simulink model "Angle_from_mpu6050_example"  (R2020b)
settings: Solver=FixedStepAuto  StartTime=0.0  StopTime=inf  RelTol=1e-3
libraries: arduinosensorlib x1
settings Model: SILPILModeSetting=veronly  ExtModeTrigDuration=2  Creator=Abdou  LastModifiedBy=Abdou
settings OptimizationCC: EnhancedBackFolding=on  PassReuseOutputArgsAs=Individual arguments  ZeroExternalMemoryAtStartup=off  ZeroInternalMemoryAtStartup=off  MaxStackSize=64  OptimizeBlockOrder=speed  DifferentSizesBufferReuse=on  OptimizationCustomize=off  EfficientTunableParamExpr=on
settings DebuggingCC: ParameterTunabilityLossMsg=error
settings HardwareCC: ProdBitPerInt=16  ProdBitPerPointer=16  ProdBitPerSizeT=16  ProdBitPerPtrDiffT=16  ProdLargestAtomicFloat=None  ProdWordSize=8  ProdHWDeviceType=Atmel->AVR
settings SFSimCC: MATLABDynamicMemAlloc=off
settings RTWCC: Description=Embedded Coder  SystemTargetFile=ert.tlc  HardwareBoard=Arduino Uno  TemplateMakefile=ert_default_tmf  Toolchain=Arduino AVR
settings CodeAppCC: ForceParamTrailComments=on  IgnoreCustomStorageClasses=off  OperatorAnnotations=on  SimulinkDataObjDesc=on  SFDataObjDesc=on  InsertBlockDesc=on
settings ERTTargetCC: SupportContinuousTime=on  SupportVariableSizeSignals=on  ExtMode=on  ExtModeStaticAllocSize=250  ExtModeMexArgs='127.0.0.1' 0 17725

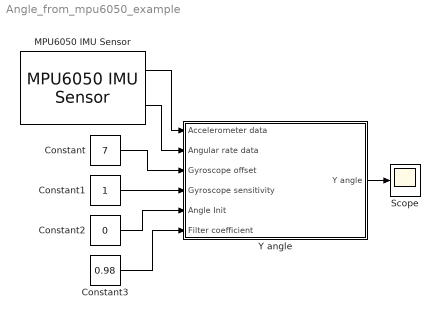
== system Angle_from_mpu6050_example ==
  Constant : Constant  Value=7
  Constant1 : Constant
  Constant2 : Constant  Value=0
  Constant3 : Constant  Value=0.98
  MPU6050 IMU Sensor : arduinosensorlib/MPU6050 IMU Sensor  SlaveAddress=0x68  Accel=on  AngularRate=on  Temperature=off  Status=off  EulerAngles=off  Quat=off  AccelRange=2G  GyroRange=250 dps  DmpOdr=200 Hz  Dlpf=Accelerometer: 5Hz, Gyroscope: 5Hz  SampleTime=1/100
      settings: SourceProductBaseCode=ARDUINO
  Scope : Scope
  Y angle : Subsystem
  wires:
  MPU6050 IMU Sensor/1 -> Y angle/1(Accelerometer data)
  MPU6050 IMU Sensor/2 -> Y angle/2(Angular rate data)
  Constant/1 -> Y angle/3(Gyroscope offset)
  Constant1/1 -> Y angle/4(Gyroscope sensitivity)
  Constant2/1 -> Y angle/5(Angle Init)
  Constant3/1 -> Y angle/6(Filter coefficient)
  Y angle/1(Y angle) -> Scope/1

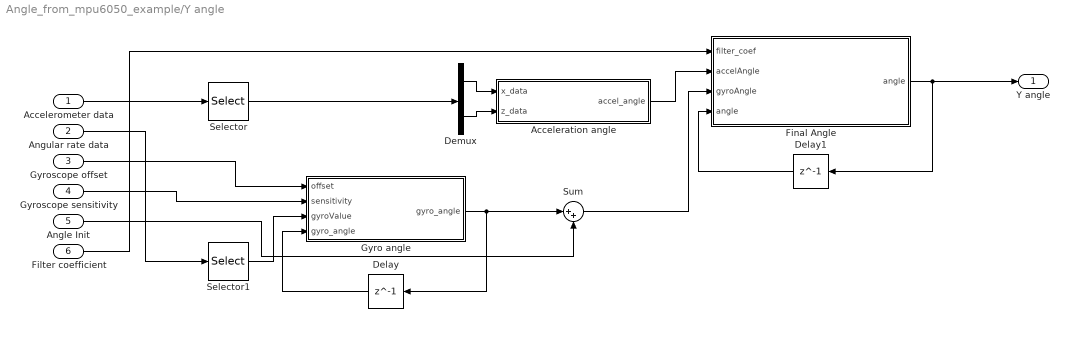
== system Angle_from_mpu6050_example/Y angle ==
  Accelerometer data : Inport
  Angular rate data : Inport  Port=2
  Gyroscope offset : Inport  Port=3
  Gyroscope sensitivity : Inport  Port=4
  Angle Init : Inport  Port=5
  Filter coefficient : Inport  Port=6
  Acceleration angle : MATLAB Function  TreatAsAtomicUnit=on
  Delay : Delay  DelayLength=1  InitialCondition=0
  Delay1 : Delay  DelayLength=1  InitialCondition=0
  Demux : Demux  Outputs=2
  Final Angle : MATLAB Function  TreatAsAtomicUnit=on
  Gyro angle : MATLAB Function  TreatAsAtomicUnit=on
  Selector : Selector  InputPortWidth=3  IndexOptions=Index vector (dialog)  Indices=[1 3]  OutputSizes=1
  Selector1 : Selector  InputPortWidth=3  IndexOptions=Index vector (dialog)  Indices=2  OutputSizes=1
  Sum : Sum  Inputs=|++
  Y angle : Outport
  wires:
  Demux/1 -> Acceleration angle/1(x_data)
  Sum/1 -> Final Angle/3(gyroAngle)
  Delay/1 -> Gyro angle/4("gyro_angle ")
  Angle Init/1 -> Sum/2
  Demux/2 -> Acceleration angle/2(z_data)
  Gyro angle/1(gyro_angle) -> Sum/1, Delay/1
  Selector1/1 -> Gyro angle/3(gyroValue)
  Final Angle/1(angle) -> Y angle/1, Delay1/1
  Filter coefficient/1 -> Final Angle/1(filter_coef)
  Selector/1 -> Demux/1
  Acceleration angle/1(accel_angle) -> Final Angle/2(accelAngle)
  Delay1/1 -> Final Angle/4("angle ")
  Gyroscope sensitivity/1 -> Gyro angle/2(sensitivity)
  Accelerometer data/1 -> Selector/1
  Angular rate data/1 -> Selector1/1
  Gyroscope offset/1 -> Gyro angle/1(offset)

== matlab function Angle_from_mpu6050_example/Y angle/Acceleration angle ==
  data: x_data input; z_data input; accel_angle output
function accel_angle = Accel_angle(x_data,z_data)
    accel_angle = atan2(x_data,z_data) * 180/pi ;

== matlab function Angle_from_mpu6050_example/Y angle/Final Angle ==
  data: filter_coef input; accelAngle input; gyroAngle input; angle output; angle input
function angle = Complimentary_filter(filter_coef,accelAngle,gyroAngle,angle)
    angle = filter_coef * (angle + gyroAngle / 100 ) + (1 - filter_coef) * accelAngle;

== matlab function Angle_from_mpu6050_example/Y angle/Gyro angle ==
  data: offset input; sensitivity input; gyroValue input; gyro_angle output; gyro_angle input
function gyro_angle = Gyro_angle(offset,sensitivity,gyroValue,gyro_angle)
    gyroRate = (gyroValue - offset) * sensitivity;
    gyro_angle = gyro_angle - gyroRate / 100.0;
